simulink model "SimulinkOnramp"  (R2026a)
settings: Solver=VariableStepAuto
StartFcn:
  | learning.simulink.modelCallbacks.startFunction(gcs);
StopFcn:
  | learning.simulink.modelCallbacks.stopFunction(gcs);
model workspace (MAT data in the model file):
  courseObject.course = 'simulink'
  courseObject.chapter = 1
  courseObject.lesson = 2
  courseObject.section = 1
  courseObject.task = 1
  t_ans = [0; 2.04842930194e-05; 0.000122905758117; 0.000635013083603; 0.00319554971103; 0.0159982328482; 0.080011648534; 0.280011648534; 0.480011648534; 0.680011648534; 0.880011648534; 1.08001164853; 1.28001164853; 1.48001164853; 1.68001164853; 1.88001164853; 2.08001164853; 2.28001164853; 2.48001164853; 2.68001164853; 2.88001164853; 3.08001164853; 3.28001164853; 3.48001164853; 3.68001164853; 3.88001164853; 4.08001164853; 4.28001164853; 4.48001164853; 4.68001164853; 4.88001164853; 5.08001164853; 5.28001164853; 5.48001164853; 5.68001164853; 5.88001164853; 6.08001164853; 6.28001164853; 6.48001164853; 6.68001164853; 6.88001164853; 7.08001164853; 7.28001164853; 7.48001164853; 7.68001164853; 7.88001164853; 8.08001164853; 8.28001164853; 8.48001164853; 8.68001164853; 8.88001164853; 9.08001164853; 9.28001164853; 9.48001164853; 9.68001164853; 9.88001164853; 10]
  y_ans1 = [0; -0.000200950914507; -0.00120570548415; -0.00622947793943; -0.0313482903266; -0.156936097029; -0.784093729248; -2.71223370643; -4.5391876483; -6.20847064999; -7.68378887699; -8.94983343311; -10.0091155707; -10.8767790245; -11.5752074514; -12.1295643539; -12.5646812012; -12.9032213047; -13.1648259152; -13.3659132186; -13.5198555134; -13.6373395062; -13.7267867214; -13.7947647461; -13.8463555711; -13.8854687081; -13.9150985117; -13.9375308341; -13.9545063252; -13.9673479832; -13.9770599428; -13.9844035116; -13.9899554273; -13.9941523378; -13.9973246769; -13.9997224142; -14.001534599; -14.0029041791; -14.0039392268; -14.0047214381; -14.0053125654; -14.0057592827; -14.0060968656; -14.0063519743; -14.0065447569; -14.0066904399; -14.00680053; -14.006883723; -14.0069465903; -14.0069940978; -14.0070299982; -14.0070571273; -14.0070776281; -14.0070931201; -14.0071048271; -14.0071136738; -14.0071179068]
  y_ans2 = [0; -0.000200950914493; -0.00120570548117; -0.00622947752872; -0.0313482379881; -0.156929530477; -0.783275242408; -2.67858776934; -4.38351296914; -5.81684912877; -6.95489131527; -7.81814270117; -8.45054140838; -8.90209881812; -9.21865994386; -9.4377357786; -9.58799561907; -9.69042408339; -9.75995470089; -9.80701922441; -9.83881526062; -9.86026815074; -9.87472975061; -9.88447267046; -9.89103394571; -9.89545138336; -9.89842492381; -9.90042627944; -9.90177319076; -9.90267961128; -9.90328957541; -9.90370003271; -9.90397623315; -9.90416208882; -9.90428715041; -9.90437130346; -9.90442792924; -9.90446603211; -9.90449167107; -9.9045089232; -9.90452053192; -9.90452834328; -9.90453359943; -9.90453713622; -9.90453951608; -9.90454111745; -9.90454219499; -9.90454292005; -9.90454340794; -9.90454373623; -9.90454395713; -9.90454410577; -9.90454420579; -9.90454427309; -9.90454431838; -9.90454434885; -9.90454436211]
libraries: signalChecks x1
CloseFcn:
  | learning.simulink.cleanupOnlineTraining;learning.simulink.Application.getInstance().dduxLogMatlabEvent("ModelClosed");
Description:
  | TrainingCourseModel
settings Model: Creator=SPARTAN PC  LastModifiedBy=SPARTAN PC

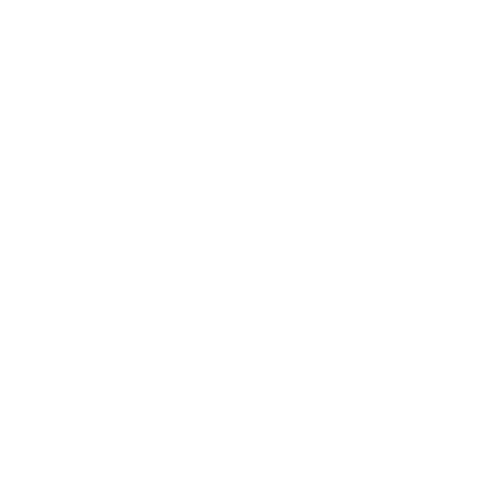
[thumbnail: Simulink's stored preview of the top-level diagram]
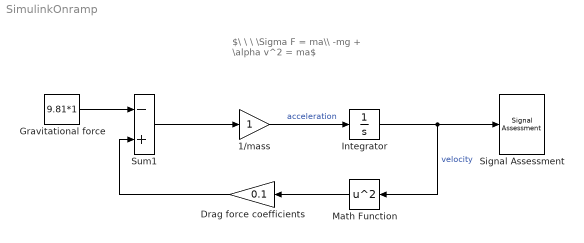
== system SimulinkOnramp ==
  note: $\ \ \ \Sigma F = ma\\ -mg + \alpha v^2 = ma$
  1/mass : Gain
  Drag force coefficients : Gain  Gain=0.1
  Gravitational force : Constant  Value=9.81*1
  Integrator : Integrator
  Math Function : Math  Operator=square  SignedPower=on
  Signal Assessment : signalChecks/Signal Assessment  signal_type='signal'  t_ans=t_ans  y_ans_upper=y_ans2  y_ans_lower=0  range=.05  rate_type=0  lesson=0  task=2  pass=1
  Sum1 : Sum  Inputs=-+
  wires:
  Sum1/1 -> 1/mass/1
  Gravitational force/1 -> Sum1/1
  Integrator/1 -> Signal Assessment/1, Math Function/1  "velocity"
  Math Function/1 -> Drag force coefficients/1
  Drag force coefficients/1 -> Sum1/2
  1/mass/1 -> Integrator/1  "acceleration"
